simulink model "Simulink_Model"  (R2021a)
settings: Solver=VariableStepAuto  StartTime=0.0  StopTime=inf  FixedStep=1  RelTol=1e-3
model workspace (MAT data in the model file):
  M = 1200
  R = 1
libraries: pid_lib x1
settings Model: EnablePacing=on  Creator=matteopenlington  LastModifiedBy=matteopenlington
settings DebuggingCC: UnderSpecifiedDimensionMsg=warning

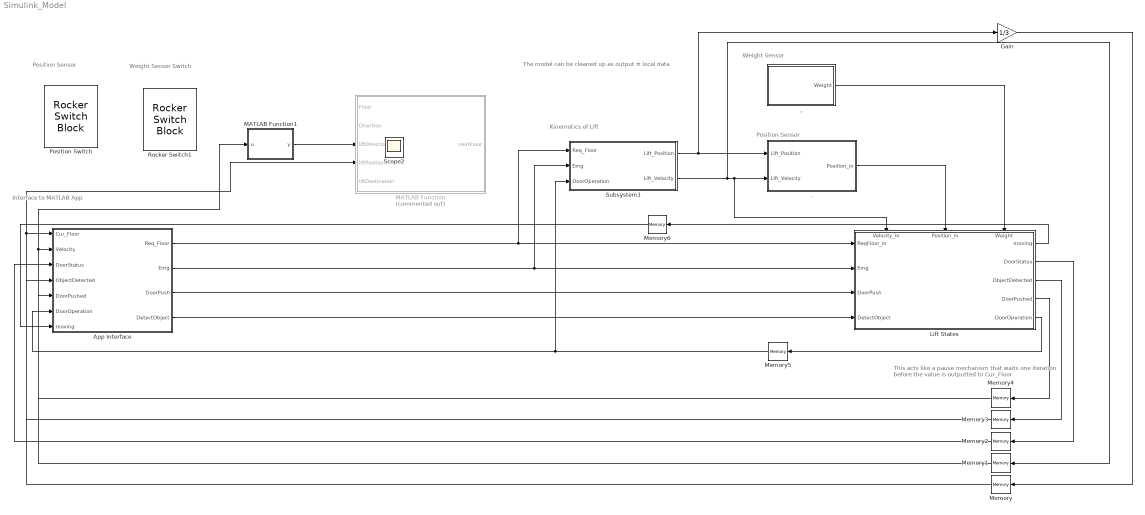
== system Simulink_Model ==
  note: Position Sensor
  note: Position Sensor
  note: Weight Sensor Switch
  note: Weight Sensor
  note: This acts like a pause mechanism that
      | waits one iteration before the value is
      | outputted to Cur_Floor
  note: The model can be cleaned up as output = local data
  note: Interface to MATLAB App
  note: Kinematics of Lift
  , : Subsystem
  . : Subsystem
  App Interface : Stateflow chart  TreatAsAtomicUnit=on
  Gain : Gain  Gain=1/3
  Lift States : Stateflow chart  TreatAsAtomicUnit=on
      settings: PortSchema="{\"entries\":[{\"content\":{\"sides\":[{\"content\":{\"connectorIds\":[\"In1\",\"In3\",\"In4\",\"In5\"]},\"type\":\"ConnectorPlacement.EquallySpacedRectSide\",\"uuid\":\"bd67e075-ced7-4894-beb9-3d24b34d513a\"},{\"content\":{\"connectorIds\":[\"Out1\",\"Out2\",\"Out3\",\"Out4\",\"Out5\"],\"side\":\"RIGHT\"},\"type\":\"ConnectorPlacement.EquallySpacedRectSide\",\"uuid\":\"62974800-2f1d-440c-84a5-b13d0b321f49\"},{\"content\":{\"connectorIds\":[\"In7\",\"In6\",\"In2\"],\"side\":\"TOP\"},\"type\":\"ConnectorPlacement.EquallySpacedRectSide\",\"uuid\":\"b0ebe389-7aaa-432d-aca6-247e3589a149\"}]},\"type\":\"ConnectorPlacement.EquallySpacedConnector\",\"uuid\":\"bed4184c-0ba6-4939-b370-ce80092994a7\"}],\"packageUris\":[\"http://schema.mathworks.com/mf0/Connector/R2020b\"],\"version\":\"1.0\"}"
  MATLAB Function : MATLAB Function  Commented=on  TreatAsAtomicUnit=on
  MATLAB Function1 : MATLAB Function  TreatAsAtomicUnit=on
  Memory{,1..6} (7 alike) : Memory
  Position Switch : RockerSwitchBlock
      settings: Values={{'Off', 'On'}, [0 1]}
  Rocker Switch1 : RockerSwitchBlock
      settings: Values={{'Off', 'On'}, [0 1]}
  Subsystem1 : Subsystem
  Scope2 : Scope
  wires:
  Memory/1 -> MATLAB Function/4(liftPosition), App Interface/1(Cur_Floor)
  Gain/1 -> Memory/1
  App Interface/2(Emg) -> Subsystem1/2(Emg), Lift States/3(Emg)
  Memory1/1 -> MATLAB Function1/1(u), App Interface/2(Velocity)
  App Interface/3(DoorPush) -> Lift States/4(DoorPush)
  Lift States/2(DoorStatus) -> Memory2/1
  Memory2/1 -> App Interface/3(DoorStatus)
  Subsystem1/2(Lift_Velocity) -> ./2(Lift_Velocity), Lift States/7(Velocity_in), Memory1/1
  App Interface/4(DetectObject) -> Lift States/5(DetectObject)
  App Interface/1(Req_Floor) -> Subsystem1/1(Req_Floor), Lift States/1(ReqFloor_in)
  Lift States/3(ObjectDetected) -> Memory3/1
  Memory3/1 -> App Interface/4(ObjectDetected)
  ./1(Position_in) -> Lift States/6(Position_in)
  Lift States/4(DoorPushed) -> Memory4/1
  Memory4/1 -> App Interface/5(DoorPushed)
  Subsystem1/1(Lift_Position) -> ./1(Lift_Position), Gain/1
  ,/1(Weight) -> Lift States/2(Weight)
  Lift States/5(DoorOperation) -> Memory5/1
  Memory5/1 -> App Interface/6(DoorOperation), Subsystem1/3(DoorOperation)
  Lift States/1(moving) -> Memory6/1
  Memory6/1 -> App Interface/7(moving)
  MATLAB Function1/1(y) -> MATLAB Function/3(liftDirection)

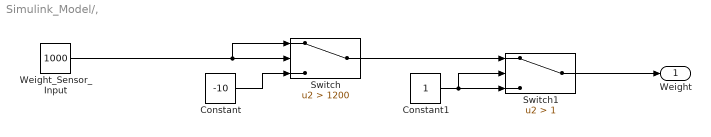
== system Simulink_Model/, ==
  Constant : Constant  Value=-10
  Constant1 : Constant
  Switch : Switch  Criteria=u2 > Threshold  Threshold=1200
  Switch1 : Switch  Criteria=u2 > Threshold  Threshold=1
  Weight_Sensor_Input : Constant  Value=1000
  Weight : Outport
  wires:
  Weight_Sensor_Input/1 -> Switch/1, Switch/2
  Switch/1 -> Switch1/1
  Constant/1 -> Switch/3
  Constant1/1 -> Switch1/3, Switch1/2
  Switch1/1 -> Weight/1

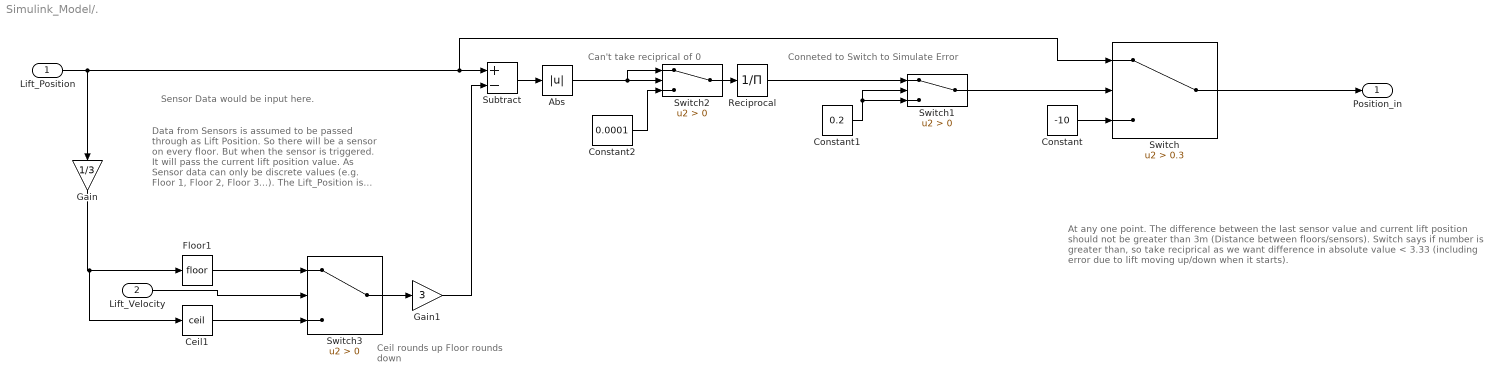
== system Simulink_Model/. ==
  note: Can't take reciprical of 0
  note: At any one point. The difference between the last sensor value and current lift position should not be greater than 3m (Distance between floors/sensors).
      |
      | Switch says if number is greater than, so take reciprical as we want difference in absolute value < 3.33 (including error due to lift moving up/down when it starts).
  note: Ceil rounds up
      | Floor rounds down
  note: Data from Sensors is assumed to be passed through as Lift Position. So there will be a sensor on every floor. But when the sensor is triggered. It will pass the current lift position value.
      |
      | As Sensor data can only be discrete values (e.g. Floor 1, Floor 2, Floor 3...). The Lift_Position is rounded to the integer according to whether velocity is up or down, as the opposite will be where the last stop was.
  note: Sensor Data would be input here.
  note: Conneted to Switch to Simulate Error
  Lift_Position : Inport
  Lift_Velocity : Inport  Port=2
  Abs : Abs
  Ceil1 : Rounding  Operator=ceil
  Constant : Constant  Value=-10
  Constant1 : Constant  Value=0.2
  Constant2 : Constant  Value=0.0001
  Floor1 : Rounding
  Gain : Gain  Gain=1/3
  Gain1 : Gain  Gain=3
  Reciprocal : Product  Inputs=/
  Subtract : Sum  Inputs=+-
  Switch : Switch  Criteria=u2 > Threshold  Threshold=0.3
  Switch1 : Switch  Criteria=u2 > Threshold
  Switch2 : Switch  Criteria=u2 > Threshold
  Switch3 : Switch  Criteria=u2 > Threshold
  Position_in : Outport
  wires:
  Lift_Position/1 -> Subtract/1, Switch/1, Gain/1
  Subtract/1 -> Abs/1
  Constant/1 -> Switch/3
  Switch/1 -> Position_in/1
  Switch1/1 -> Switch/2
  Abs/1 -> Switch2/1, Switch2/2
  Constant1/1 -> Switch1/3, Switch1/2
  Lift_Velocity/1 -> Switch3/2
  Switch3/1 -> Gain1/1
  Floor1/1 -> Switch3/1
  Ceil1/1 -> Switch3/3
  Gain/1 -> Floor1/1, Ceil1/1
  Gain1/1 -> Subtract/2
  Constant2/1 -> Switch2/3
  Switch2/1 -> Reciprocal/1
  Reciprocal/1 -> Switch1/1

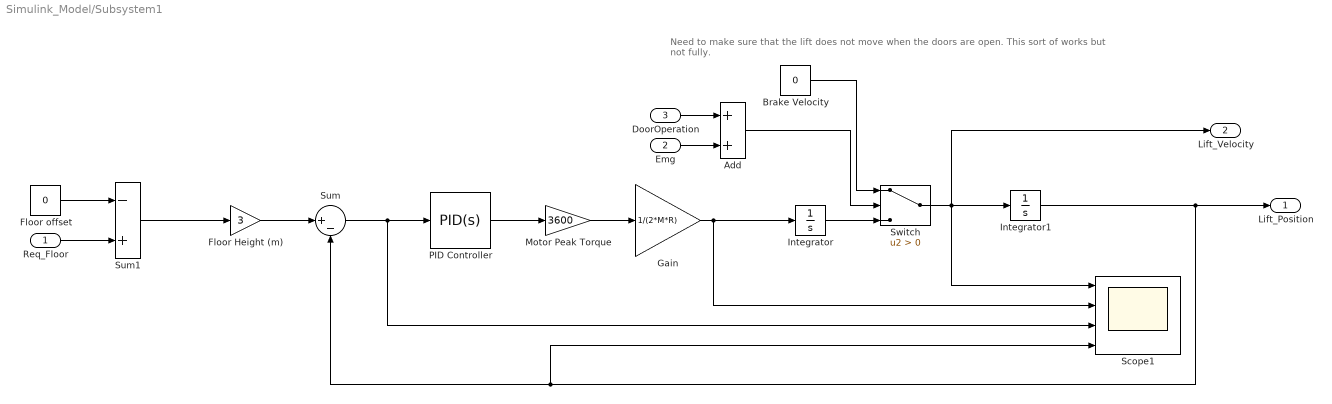
== system Simulink_Model/Subsystem1 ==
  note: Need to make sure that the lift does not move when the doors are open. This sort of works but not fully.
  Req_Floor : Inport
  Emg : Inport  Port=2
  DoorOperation : Inport  Port=3
  Add : Sum
  Brake Velocity : Constant  Value=0
  Floor Height (m) : Gain  Gain=3
  Floor offset : Constant  Value=0
  Gain : Gain  Gain=1/(2*M*R)
  Integrator : Integrator
  Integrator1 : Integrator
  Motor Peak Torque : Gain  Gain=3600
  PID Controller : pid_lib/PID Controller  Controller=PID  Form=Parallel  TimeDomain=Continuous-time  UseExternalTs=off  SampleTime=-1  IntegratorMethod=Forward Euler  FilterMethod=Forward Euler  ControllerParametersSource=internal  P=1  I=0  D=2  UseFilter=on  N=5.45  TunerSelectOption=Transfer Function Based (PID Tuner App)  InitialConditionSource=internal  InitialConditionForIntegrator=0  InitialConditionForFilter=0  DifferentiatorICPrevScaledInput=0  ExternalReset=none  TrackingMode=off  Kt=1  LimitOutput=on  SatLimitsSource=internal  UpperSaturationLimit=1  LowerSaturationLimit=-1  LinearizeAsGain=on  AntiWindupMode=none  Kb=1  POutMin=[]  POutMax=[]  IOutMin=[]  IOutMax=[]  DOutMin=[]  DOutMax=[]  NOutMin=[]  NOutMax=[]  SumOutMin=[]  SumOutMax=[]  SaturationOutMin=[]  SaturationOutMax=[]  PParamMin=[]  PParamMax=[]  IParamMin=[]  IParamMax=[]  DParamMin=[]  DParamMax=[]  NParamMin=[]  NParamMax=[]  KbParamMin=[]  KbParamMax=[]  KtParamMin=[]  KtParamMax=[]  KbOutMin=[]  KbOutMax=[]  KtOutMin=[]  KtOutMax=[]  IntegratorOutMin=[]  IntegratorOutMax=[]  FilterOutMin=[]  FilterOutMax=[]  SumI1OutMin=[]  SumI1OutMax=[]  SumI2OutMin=[]  SumI2OutMax=[]  SumI3OutMin=[]  SumI3OutMax=[]  SumI4OutMin=[]  SumI4OutMax=[]  SumDOutMin=[]  SumDOutMax=[]  DifferentiatorOutMin=[]  DifferentiatorOutMax=[]  FilterDiffOutCoefMin=[]  FilterDiffOutCoefMax=[]  ReciprocalOutMin=[]  ReciprocalOutMax=[]  SumDenOutMin=[]  SumDenOutMax=[]  SumNumOutMin=[]  SumNumOutMax=[]  DivideOutMin=[]  DivideOutMax=[]  UdiffTsProdOutMin=[]  UdiffTsProdOutMax=[]  NTsProdOutMin=[]  NTsProdOutMax=[]  UintegralTsProdOutMin=[]  UintegralTsProdOutMax=[]  UngainTsProdOutMin=[]  UngainTsProdOutMax=[]  IntegratorContinuousStateAttributes=''  IntegratorStateMustResolveToSignalObject=off  IntegratorRTWStateStorageClass=Auto  FilterContinuousStateAttributes=''  FilterStateMustResolveToSignalObject=off  FilterRTWStateStorageClass=Auto  ParallelPVariant=InternalParameters  IdealPVariant=Disabled  IVariant=InternalParameters  DVariant=InternalParameters  IntegratorVariant=Continuous  SatVariant=Enabled  AWVariant=Passthrough  PCopyVariant=Disabled  TRVariant=Disabled  FdbkBlocksVariant=Forward  IdealPFdbkVariant=Disabled  SatFdbkVariant=Disabled  DerivativeFilterVariant=ContFilter  NVariant=InternalParameters  NCopyVariant=Disabled  FilterICVariant=InternalICsFilter  IntegratorICVariant=InternalICs  ExternalResetVariant=Disabled  TRSumVariant=Passthrough  SumFdbkVariant=Disabled  SumVariant=Sum_PID  TsampFilterVariant=InternalTs  TsampNgainVariant=Passthrough  TsampIntegralVariant=Passthrough  ExternalSaturationOutDataTypeStr=Inherit: Same as second input
  Scope1 : Scope  NumInputPorts=4
  Sum : Sum  Inputs=|+-
  Sum1 : Sum  Inputs=-+
  Switch : Switch  Criteria=u2 > Threshold
  Lift_Position : Outport
  Lift_Velocity : Outport  Port=2
  wires:
  Req_Floor/1 -> Sum1/2
  Gain/1 -> Scope1/2, Integrator/1
  Sum/1 -> Scope1/3, PID Controller/1
  PID Controller/1 -> Motor Peak Torque/1
  Floor Height (m)/1 -> Sum/1
  Sum1/1 -> Floor Height (m)/1
  Integrator/1 -> Switch/3
  Integrator1/1 -> Lift_Position/1, Scope1/4, Sum/2
  Motor Peak Torque/1 -> Gain/1
  Floor offset/1 -> Sum1/1
  Switch/1 -> Scope1/1, Lift_Velocity/1, Integrator1/1
  Brake Velocity/1 -> Switch/1
  Emg/1 -> Add/2
  DoorOperation/1 -> Add/1
  Add/1 -> Switch/2

== stateflow chart Simulink_Model/App Interface ==
  state InterfaceFromApp
    en:
    coder.extrinsic('AppWSimulink', 'updateCounter', 'Logic', 'Emergency', 'DoorOperationReq', 'updateDoorStatus');
    app = AppWSimulink(this);
    %Req_Floor = 2;
    initialiseData();
    Logic(app,Req_Floor);
    Emergency(app,Emg);
    DoorOperationReq(app, DoorPush)
    du:
    if hasChanged(Cur_Floor)
    updateCounter(app, Cur_Floor, moving, DoorOperation);
    end
    if abs(Req_Floor - Cur_Floor) < 0.1
    updateDoorStatus(app,DoorStatus, ObjectDetected);
    end
    if (Emg == 1)
    Reset;
    end
    if DoorPushed == 1
    DoorPush = -2;
    end
    state initialiseData [function]
      (default) -> (junction 12) : {
          | %CurFloor = 0;
          | Req_Floor = 0;
          | Emg = 0;
          | DoorPush =-2;
          | DetectObject =-1 ;
          | }
    state Reset [function]
      (default) -> (junction 119) : {
          | Req_Floor = Cur_Floor;
          | DoorPush =3;
          | }
  (default) -> InterfaceFromApp
  data: app local; Cur_Floor input; Req_Floor output; Emg output; Velocity input; DoorPush output; DoorStatus input; DetectObject output; ObjectDetected input; DoorPushed input; DoorOperation input; moving input

== stateflow chart Simulink_Model/Lift States ==
  state No_Error2
    entry:
    door = 0;
    doorClose = 0;
    DoorStatus = 3;
    hasOpened = 1;
    DoorPushed = 0;
    DoorOperation = 0;
    state Motion [group]
      state MovingUp
        entry:
        moving = 1;
        exit:
        moving = 0;
      state MovingDown
        entry:
        moving = 2;
        exit:
        moving =0;
    state Not_Moving
      entry:
      Cur_Floor;
      NxtFloor;
      ObjectDetected = -1;
      state NxtFloor [function]
        (default) -> (junction 212)
        (junction 212) -> (junction 213) [order 1] : [isempty(ReqFloor_in)]{ReqFloor = -10}
        (junction 212) -> (junction 214) [order 2] : {ReqFloor = ReqFloor_in;}
        (junction 213) -> (junction 215)
        (junction 214) -> (junction 215)
      state Idle
        en:
      state Doors
        state OpOpening [function]
          note: If the door movement was simulated that value would end up being exactly 0 or 1. Because of step iterations you end up with 1.1 and -0.1. But the transitions account for this.
          (default) -> (junction 231) : [door <= 1]{door = door + 0.1;}
        note: Value of door isn't always 0 or 1
        state OpClosing [function]
          (default) -> (junction 244) : {door = door - 0.1;}
        state DoorOpening
          en:
          door = 0;
          doorClose = 0;
          DoorStatus = 0;
          du:
          OpOpening;
        state ObjectDetection [function]
          (default) -> (junction 290)
          (junction 290) -> (junction 292) [order 1] : [DetectObject ==1]{ObjectDetected = 1;}
          (junction 290) -> (junction 294) [order 2] : {ObjectDetected = 0;}
          (junction 292) -> (junction 297)
          (junction 294) -> (junction 297)
        state DoorClosing
          en:
          DoorStatus = 2;
          DoorPushed = 0;
          du:
          ObjectDetection;
          OpClosing;
        state DoorOpen
          entry:
          DoorStatus = 1;
          hasOpened = 1;
        state DoorClosed
          entry:
          DoorStatus =3;
          pause(2);
          doorClose = 1;
        (junction 318) -> DoorOpening
        DoorClosing -> (junction 318) [order 1] : [ObjectDetected == 1]
        (junction 321) -> DoorOpening
        DoorClosing -> (junction 321) [order 2] : [DoorPush == 0]{DoorPushed = 1;}
        DoorOpening -> DoorOpen : [door >= 1]{DoorPushed = 0;}
        DoorOpen -> DoorClosing [order 2] : [DoorPush == 1]{DoorPushed = 1;}
        DoorClosing -> DoorClosed [order 3] : [door <= 0]
        DoorOpen -> DoorClosing [order 1] : after(2,sec)
      (default) -> Idle
      Idle -> DoorOpening [order 1] : [ (ReqFloor - CurFloor)<0.01 && hasOpened == 0]{DoorOperation =1;}
    state Cur_Floor [function]
      (default) -> (junction 279) : {CurFloor = (Position_in/3);}
    note: Set DoorPush == -2 because it has been completed. But don't want to set ObjectDetected == 0 because we need to run again and make sure there are no objects in the way.
    (default) -> Not_Moving
    Not_Moving -> MovingUp [order 1] : [Velocity_in > 0.2 && DoorOperation == 0]{hasOpened = 0;}
    MovingUp -> Not_Moving : [abs(Velocity_in) < 0.01]
    Idle -> (junction 192) [order 2]
    (junction 192) -> (junction 193)
    Not_Moving -> MovingDown [order 2] : [Velocity_in < -0.2 && DoorOperation == 0]{hasOpened = 0;}
    (junction 193) -> Not_Moving : after(1,sec)
    (junction 194) -> (junction 193)
    MovingDown -> Not_Moving : [abs(Velocity_in) < 0.01]
    Doors -> (junction 194) : [doorClose == 1]{DoorOperation = 0;}
  state Error_States
    en:
    state Emergency
      en:
      DoorStatus = 0;
      hasOpened = 0;
      moving = 0;
    state Position_Sensor
      en:
      DoorStatus = 0;
      hasOpened = 0;
      moving = 0;
    state Weight_Limit
      % call to intercom to say passengers need to get off.
      en:
      DoorStatus = 0;
      hasOpened = 0;
      moving = 0;
  (default) -> No_Error2
  No_Error2 -> Emergency [order 1] : [Emg == 1]
  Emergency -> No_Error2 : [Emg  == 0]
  No_Error2 -> Position_Sensor [order 2] : [Position_in == -10]
  Position_Sensor -> No_Error2 : [Position_in~= -10]
  No_Error2 -> Weight_Limit [order 3] : [Weight == -10]
  Weight_Limit -> No_Error2 : [Weight ~= -10]
  data: CurFloor local; ReqFloor_in input; Weight input; ReqFloor local; Emg input; moving output =0; DoorPush input; DetectObject input; door local; DoorStatus output; hasOpened local; doorClose local; Position_in input; Velocity_in input; ObjectDetected output; Passengers local; DoorPushed output; DoorOperation output

== matlab function Simulink_Model/MATLAB Function ==
  data: Floor input; nextFloor output; Direction input; liftDirection input; liftPosition input; liftDestination input
function nextFloor = liftCall(Floor, Direction, liftDirection, liftPosition, liftDestination)
%% Init. Variables and Data
global passengerMatrix
passengerMatrix = []; % 2D Array

global maxPassengers
maxPassengers = 10;

%% Lift Request Button Pressed
function nextFloor = liftCall(Floor,Direction,liftDirection,liftPosition,liftDestination) % nextFloor changes from existing if redirection to be done
    % Generates New User ID in the Passenger Matrix
    avgFloor = 0;
    if Direction == "Up"
        avgFloor = round(((10 - Floor)/2) + Floor);
    else
        avgFloor = round(Floor / 2);
    end
    
    passenger = [double(Floor), now, avgFloor, 0, 0, Direction];
    
    global passengerMatrix % Adds to Passenger Matrix, also checks if empty
    if size(passengerMatrix,1) == 0
        passengerMatrix = passenger;
    else
        passengerMatrix = [passengerMatrix; passenger];
    end
    
    % Checks if request is en-route and that there is no urgent passenger
    
    overtimeFloor = overtimeCheck();
    
    nextFloor = 0;
    
    if double(overtimeFloor) ~= 0
        if liftDirection == "Up" && overtimeFloor > liftPosition && overtimeFloor < liftDestination
            nextFloor = overtimeFloor;
        elseif liftDirection == "Down" && overtimeFloor < liftPosition && overtimeFloor > liftDestination
            nextFloor = overtimeFloor;
        else
            nextFloor = liftDestination;
        end
    else
        if liftDirection == "None" % Lift is Stationary
            nextFloor = Floor;
        elseif liftDirection == "Up" && Floor > liftPosition && Direction == liftDirection && Floor < liftDestination
            nextFloor = Floor;
        elseif liftDirection == "Down" && Floor < liftPosition && Direction == liftDirection && Floor > liftDestination
            nextFloor = Floor;
        else
            nextFloor = liftDestination;
        end
    end  
    
    % Checks if doing the re-route will cause too many passengers to be
    % picked up
    global maxPassengers
    if nextFloor == Floor
        tempCounter = 0
        currentPassengers = 0
        for j = 1:size(passengerMatrix,1)
            passengerMatrix(j,4)
            if double(passengerMatrix(j,4)) ~= 0
                currentPassengers = currentPassengers + 1
            end
            if double(passengerMatrix(j,5)) == Floor
                tempCounter = tempCounter - 1
            elseif double(passengerMatrix(j,1)) == Floor
                tempCounter = tempCounter + 1
            end
        end
        if currentPassengers + tempCounter > maxPassengers
            nextFloor = liftDestination;
        end
    end
        
    
    %Check if enough time to slow down
    function bestNextFloor = liftStopped(liftFloor, buttonPressed)% buttonPressed = Internal Button
        global passengerMatrix;

        % Checks for passengers getting off on this floor, and assinging floors
        % to passengers getting on at the floor
        buttonPressedTemp = buttonPressed;
        allocationCounter = 1;
        tempCounter = size(passengerMatrix,1)
        i = 1;
        while i <= tempCounter % goes through passenger matrix
            if double(passengerMatrix(i,5)) == liftFloor
                passengerMatrix(i,:) = []; % Deletes from Passenger Matrix if they got off here
                tempCounter = tempCounter - 1
            elseif double(passengerMatrix(i,1)) == liftFloor && double(passengerMatrix(i,4)) == 0
                passengerMatrix(i,4) = now; % Adds wait time to Passenger Matrix if they got on here
                passengerMatrix(i,5) = buttonPressedTemp(allocationCounter); %appends actual floor to person who got on here
                if allocationCounter < length(buttonPressed) % Checks if multiple floor buttons pressed
                    allocationCounter = allocationCounter + 1; % as buttonPressed can be array, work through the list
                end
                i = i + 1;
            else
                i = i + 1;
            end
        end


        stopArray = [];
        motionArray = [];

        pickupArray = [];
        distinationArray = [];
        directionArray = [];
        passengerDone = [];
        for i = 1:size(passengerMatrix,1) % Goes through passenger matrix
            pickupArray(i) = passengerMatrix(i,1); % Pickup location
            if double(passengerMatrix(i,5)) == 0
                destinationArray(i) = passengerMatrix(i,3); % Dropoff Location (ESTIMATED)
            else
                destinationArray(i) = passengerMatrix(i,5); % Dropoff Location (ACTUAL)
            end
            directionArray = [directionArray passengerMatrix(i,6)];
            if double(passengerMatrix(i,4)) == 0
                passengerDone(i) = 1;
            else
                passengerDone(i) = 2;
            end
        end

        minPath = 0;
        timeStop = 5;
        timeMotion = 1;
        timeArrayUp = []; % Where results of Up calculation are held
        locationArrayUp = [];
        timeArrayDown = []; % Where results of Down calculation are held
        locationArrayDown = [];
        for i = 1:10 % Cycles through each floor (1-10)
            currentPath = abs(liftFloor - i)  * (length(passengerDone) - sum(passengerDone(:) == 3)) * (timeStop + timeMotion); % Cost to travel to current tested floor
            % START UP
            if i ~= 10 %Doesn't go up if on top floor
                    currentStops = 0;
                    currentMotion = 0;
                    Direction = "Up";
                    floorTemp = i;
                    flag = 0;

                    passengerDone = [];
                    for i2 = 1:size(passengerMatrix,1) % Goes through passenger matrix
                        if double(passengerMatrix(i2,4)) == 0
                            passengerDone(i2) = 1;
                        else
                            passengerDone(i2) = 2;
                        end
                    end

                    currentJobArray = [];
                    for j = 1:size(passengerMatrix,1) % Cycles through the entire passsenger matrix to check for passengers in same direction
                        if directionArray(j) == Direction
                                currentJobArray = [currentJobArray pickupArray(j)];
                                currentJobArray = [currentJobArray destinationArray(j)];
                        end
                    end

                    sortedJobs = unique(sort(double(currentJobArray))); % Sorts array and removes duplicates for Up
                    startIndex = find(double(unique(sort([currentJobArray floorTemp]))) == double(floorTemp)); %%CHANGES THESE IN BELOW FOR GOING DOWN, FLIP SORT
                    currentJobArray = [];
                    for j = 1:size(passengerMatrix,1)
                        if directionArray(j) ~= Direction
                                currentJobArray = [currentJobArray pickupArray(j)];
                                currentJobArray = [currentJobArray destinationArray(j)];
                        end
                    end

                    sortedJobs2 = fliplr(unique(sort(double(currentJobArray)))); % repeat for opposite, flipped (higher floors first)

                    % Checks the index position of the nearest demanded floor, will
                    % set that floor as the first desitination

                    inuseArray = sortedJobs;
                    locationArray = [];
                        while ismember(1,passengerDone()) == 1 || ismember(2,passengerDone()); % While there is still demand
                            global maxPassengers % Checks again for passenger overload
                            tempCounter = 0;
                            currentPassengers = 0;
                            for j = 1:size(passengerMatrix,1)
                                if double(passengerMatrix(j,4)) ~= 0
                                    currentPassengers = currentPassengers + 1;
                                end
                                startIndex
                                inuseArray
                                double(passengerMatrix(j,5))
                                if double(passengerMatrix(j,5)) == inuseArray(startIndex)
                                    tempCounter = tempCounter - 1;
                                elseif double(passengerMatrix(j,1)) == inuseArray(startIndex)
                                    tempCounter = tempCounter + 1;
                                end
                            end
                            if currentPassengers + tempCounter <= maxPassengers
                                for i2 = 1:size(passengerMatrix,1) % Checks each passenger and adjusts their current status at this gloor
                                    if directionArray(i2) == Direction
                                        if passengerDone(i2) == 1 && pickupArray(i2) == inuseArray(startIndex)
                                            passengerDone(i2) = 2;
                                            if flag ~= 1
                                                locationArray(length(locationArray) + 1) = inuseArray(startIndex);
                                                currentStops = currentStops + (1 * (length(passengerDone) - sum(passengerDone(:) == 3)));
                                                currentMotion = double(currentMotion) + (abs(double(inuseArray(startIndex)) - double(floorTemp)) * (double(length(passengerDone)) - double(sum(passengerDone(:) == 3))));
                                                floorTemp = inuseArray(startIndex);
                                                flag = 1;
                                            end
                                        end
                                        if passengerDone(i2) == 2 && double(destinationArray(i2)) == inuseArray(startIndex)
                                            passengerDone(i2) = 3;
                                            if flag ~= 1
                                                locationArray(length(locationArray) + 1) = inuseArray(startIndex);
                                                currentStops = currentStops + (1 * (length(passengerDone) - sum(passengerDone(:) == 3)));
                                                currentMotion = double(currentMotion) + (abs(double(inuseArray(startIndex)) - double(floorTemp)) * (double(length(passengerDone)) - double(sum(passengerDone(:) == 3))));
                                                floorTemp = inuseArray(startIndex);
                                                flag = 1;
                                            end
                                        end
                                    end
                                end
                            end

                            % Checks if the index position should be reset at end
                            % of floors

                            if Direction == "Up" && startIndex == length(inuseArray)
                                Direction = "Down";
                                startIndex = 0;
                                inuseArray = sortedJobs2;
                            elseif Direction == "Down" && startIndex == length(inuseArray)
                                Direction = "Up";
                                startIndex = 0;
                                inuseArray = sortedJobs;
                            end
                            startIndex = startIndex + 1;
                            flag = 0;
                        end
                timeArrayUp(length(timeArrayUp)+1) = ((currentStops * timeStop) + (currentMotion * timeMotion)) + currentPath; % Added +1
                locationArrayUp = [locationArrayUp locationArray(1)];
            end


            % START DOWN
            if i ~= 1 %Doesn't go down if on bottom floor
                    currentStops = 0;
                    currentMotion = 0;
                    Direction = "Down";
                    floorTemp = i;
                    flag = 0;

                    passengerDone = [];
                    for i2 = 1:size(passengerMatrix,1) % Goes through passenger matrix
                        if double(passengerMatrix(i2,4)) == 0
                            passengerDone(i2) = 1;
                        else
                            passengerDone(i2) = 2;
                        end
                    end

                    %passengerDone
                    currentJobArray = [];
                    for j = 1:size(passengerMatrix,1) % Cycles through the entire passsenger matrix to check for passengers in same direction
                        if directionArray(j) ~= Direction
                            currentJobArray = [currentJobArray pickupArray(j)];
                            currentJobArray = [currentJobArray destinationArray(j)];
                        end
                    end

                    sortedJobs = fliplr(unique(sort(double(currentJobArray)))); % Sorts array and removes duplicates for Down, flipped
                    startIndex = find(double(unique(sort([currentJobArray floorTemp]))) == double(floorTemp)); %%CHANGES THESE IN BELOW FOR GOING DOWN, FLIP SORT

                    currentJobArray = [];
                    for j = 1:size(passengerMatrix,1)
                        if directionArray(j) == Direction
                            currentJobArray = [currentJobArray pickupArray(j)];
                            currentJobArray = [currentJobArray destinationArray(j)];
                        end
                    end

                    sortedJobs2 = unique(sort(double(currentJobArray))); % repeat for opposite

                    % Checks the index position of the nearest demanded floor, will
                    % set that floor as the first desitination

                    inuseArray = sortedJobs;
                    locationArray = [];

                        while ismember(1,passengerDone()) == 1 || ismember(2,passengerDone()) % While there is still demand
                            global maxPassengers % Checks again for passenger overload
                            tempCounter = 0;
                            currentPassengers = 0;
                            for j = 1:size(passengerMatrix,1)
                                if double(passengerMatrix(j,4)) ~= 0
                                    currentPassengers = currentPassengers + 1;
                                end
                                if double(passengerMatrix(j,5)) == inuseArray(startIndex)
                                    tempCounter = tempCounter - 1;
                                elseif double(passengerMatrix(j,1)) == inuseArray(startIndex)
                                    tempCounter = tempCounter + 1;
                                end
                            end
                            if currentPassengers + tempCounter <= maxPassengers
                                %passengerDone
                                %inuseArray(startIndex)
                                for i2 = 1:size(passengerMatrix,1) % Checks each passenger and adjusts their current status at this gloor

                                    if directionArray(i2) == Direction
                                        if passengerDone(i2) == 1 && pickupArray(i2) == inuseArray(startIndex)
                                            passengerDone(i2) = 2;
                                            if flag ~= 1
                                                locationArray(length(locationArray) + 1) = inuseArray(startIndex);
                                                currentStops = currentStops + (1 * (length(passengerDone) - sum(passengerDone(:) == 3)));
                                                currentMotion = double(currentMotion) + (abs(double(inuseArray(startIndex)) - double(floorTemp)) * (double(length(passengerDone)) - double(sum(passengerDone(:) == 3))));
                                                floorTemp = inuseArray(startIndex);
                                                flag = 1;
                                            end
                                        end
                                        if double(passengerDone(i2)) == 2 && double(destinationArray(i2)) == inuseArray(startIndex)
                                            passengerDone(i2) = 3;
                                            if flag ~= 1
                                                locationArray(length(locationArray) + 1) = inuseArray(startIndex);
                                                currentStops = currentStops + (1 * (length(passengerDone) - sum(passengerDone(:) == 3)));
                                                currentMotion = double(currentMotion) + (abs(double(inuseArray(startIndex)) - double(floorTemp)) * (double(length(passengerDone)) - double(sum(passengerDone(:) == 3))));
                                                floorTemp = inuseArray(startIndex);
                                                flag = 1;
                                            end
                                        end
                                    end
                                end
                            else

                            end

                            % Checks if the index position should be reset at end
                            % of floors
                            if Direction == "Up" && double(startIndex) == length(inuseArray)
                                Direction = "Down";
                                startIndex = 0;
                                inuseArray = sortedJobs2;
                            elseif Direction == "Down" && double(startIndex) == length(inuseArray)
                                Direction = "Up";
                                startIndex = 0;
                                inuseArray = sortedJobs;
                            end
                            startIndex = startIndex + 1;
                            flag = 0;
                        end
                timeArrayDown(length(timeArrayDown)+1) = ((currentStops * timeStop) + (currentMotion * timeMotion)) + currentPath;
                stopArray(length(stopArray)+1) = currentStops;
                motionArray(length(motionArray)+1) = currentMotion;
                locationArrayDown = [locationArrayDown locationArray(1)];
            end
        end
        % Compares up and Down Times, picks the shortest and spits out the best next
        % floor to go to

        timeArrayUp
        timeArrayDown

        locationArrayDown
        locationArrayUp


        bestNextFloor = 0;
        sortUp = sort(timeArrayUp);
        sortDown = sort(timeArrayDown);
        if sortUp(1) < sortDown(1)
            bestNextFloor = locationArrayUp(find(timeArrayUp == sortUp(1))); % Extracts the index of the best next floor
        else
            timeArrayDown
            find(timeArrayDown == sortDown(1))
            bestNextFloor = locationArrayDown(find(timeArrayDown == sortDown(1)));
        end

        if overtimeCheck() ~= 0
            bestNextFloor = overtimeCheck();
        end
    end
    
    function priorityFloor = overtimeCheck()
        % Goes through Pass.Mtrx and checks for overtime
        global passengerMatrix
        overtimePos = [];
        overtimeWait = [];
        overtimeType = [];
        for i = 1:size(passengerMatrix,1)
            if now - double(passengerMatrix(i,2)) > 45000 && double(passengerMatrix(i,4)) == 0
                overtimePos(length(overtimePos) + 1) = i;
                overtimeWait(length(overtimeWait) + 1) = now - double(passengerMatrix(i,2)) - 45000; %Target Times in Milliseconds
                overtimeType(length(overtimePos) + 1) = "Wait";
            elseif now - double(passengerMatrix(i,4)) > 45000  && double(passengerMatrix(i,4)) ~= 0
                overtimePos(length(overtimePos) + 1) = i;
                overtimeWait(length(overtimeWait) + 1) = now - double(passengerMatrix(i,4)) - 45000;
                overtimeType(length(overtimePos) + 1) = "Lift";
            elseif ((now - (double(passengerMatrix(i,4))))+(double(passengerMatrix(i,4))-double(passengerMatrix(i,2)))) > 60000  && double(passengerMatrix(i,4)) ~= 0
                overtimePos(length(overtimePos) + 1) = i;
                overtimeWait(length(overtimeWait) + 1) = ((now - (double(passengerMatrix(i,4))))+(double(passengerMatrix(i,4))-double(passengerMatrix(i,2)))) - 60000;
                overtimeType(length(overtimePos) + 1) = "Lift";
            end
        end

        % Checks if overtime present, where to go first.

        if length(overtimeWait) > 0
            sortWaitTimes = sort(overtimeWait);
            priorityIndex = find(overtimeWait == sortWaitTimes(length(sortWaitTimes)));
            priorityFloor = passengerMatrix(overtimePos(priorityIndex),1);
        else
            priorityFloor = 0;
        end
    end
end

== matlab function Simulink_Model/MATLAB Function1 ==
  data: u input; y output
function y = fcn(u)
    if u>0
        y = "Up";
    elseif u<0
        y = "Down";
    else
        y = "None";
    end
end
